simulink model "MiniHR"  (R2023a)
settings: Solver=FixedStepAuto  StartTime=0.0  StopTime=90  RelTol=1e-3
PreLoadFcn:
  | k=0.0001;
InitFcn:
  | k=0.0001;
values from neighbouring files (symbols this model uses):
  X = T(4)    [arm_contr.m]
  Y = T(5)    [arm_contr.m]
  Z = T(6)    [arm_contr.m]
libraries: sm_lib x208, nesl_utility x28, simulink x2
(part 6 of 6)

== system MiniHR/Subsystem/right_foot_y ==
  Visual : sm_lib/Body Elements/File Solid  ExtGeomFileName=小人形关节整合02/meshes/right_foot_y.STL  UnitType=Custom  ExtGeomFileUnits=m  StepReaderType=HEX  ExportConvexHullGeometry=off  InertiaType=Custom  Mass=0.204168570722069  MassUnits=kg  CenterOfMass=[0, 0, 0]  CenterOfMassUnits=m  MomentsOfInertia=[8.623203481057019e-05, 5.19196934874567e-05, 5.75861568294968e-05]  MomentsOfInertiaUnits=kg*m^2  ProductsOfInertia=[-6.07410466001495e-10, -1.79197419171308e-07, -1.07327974268827e-09]  ProductsOfInertiaUnits=kg*m^2  BasedOnType=DensityFromFile  Density=1000  DensityUnits=kg/m^3  DoExposeReferenceFrame=on  SerializedFrames=<Frames/>  GraphicType=FromGeometry  MarkerShape=Sphere  MarkerSize=10  GraphicVisPropType=SimpleVisualProperties  GraphicDiffuseColor=[1.0 0.2 1.0]  GraphicSpecularColor=[0.5 0.5 0.5 1.0]  GraphicAmbientColor=[0.15 0.15 0.15 1.0]  GraphicEmissiveColor=[0.0 0.0 0.0 1.0]  GraphicShininess=75  GraphicOpacity=1
  VisualOriginTransform : sm_lib/Frames and Transforms/Rigid Transform  TranslationMethod=Cartesian  TranslationStandardOffset=0  TranslationStandardOffsetUnits=m  TranslationStandardAxis=+Z  TranslationCartesianOffset=[0, 0, 0]  TranslationCartesianOffsetUnits=m  TranslationROffset=0  TranslationROffsetUnits=m  TranslationZOffset=0  TranslationZOffsetUnits=m  TranslationThetaOffset=0  TranslationThetaOffsetUnits=deg  RotationMethod=RotationSequence  RotationAngleUnits=deg  RotationStandardAxis=+Z  RotationAngle=0.0  RotationArbitraryAxis=[0 0 1]  FollAlignAxisA=+X  BaseAlignAxisA=+Y  FollAlignAxisB=+Y  BaseAlignAxisB=+Z  RotationSequenceAxes=BaseAxes  RotationSequence=XYZ  RotationSequenceAngles=[0, 0, 0]  RotationSequenceAnglesUnits=rad  RotationMatrix=[1 0 0; 0 1 0; 0 0 1]  Quaternion=[1 0 0 0]
  right_foot_x_jo_AxisTransform : sm_lib/Frames and Transforms/Rigid Transform  TranslationMethod=Cartesian  TranslationStandardOffset=0  TranslationStandardOffsetUnits=m  TranslationStandardAxis=+Z  TranslationCartesianOffset=[0, 0, 0]  TranslationCartesianOffsetUnits=m  TranslationROffset=0  TranslationROffsetUnits=m  TranslationZOffset=0  TranslationZOffsetUnits=m  TranslationThetaOffset=0  TranslationThetaOffsetUnits=deg  RotationMethod=ArbitraryAxis  RotationAngleUnits=rad  RotationStandardAxis=+Z  RotationAngle=1.570796326794897  RotationArbitraryAxis=[0, -1, 0]  FollAlignAxisA=+X  BaseAlignAxisA=+Y  FollAlignAxisB=+Y  BaseAlignAxisB=+Z  RotationSequenceAxes=FollowerAxes  RotationSequence=XYX  RotationSequenceAngles=[0 0 0]  RotationSequenceAnglesUnits=deg  RotationMatrix=[1 0 0; 0 1 0; 0 0 1]  Quaternion=[1 0 0 0]
  right_foot_x_jo_OriginTransform : sm_lib/Frames and Transforms/Rigid Transform  TranslationMethod=Cartesian  TranslationStandardOffset=0  TranslationStandardOffsetUnits=m  TranslationStandardAxis=+Z  TranslationCartesianOffset=[0, 0, -0.037]  TranslationCartesianOffsetUnits=m  TranslationROffset=0  TranslationROffsetUnits=m  TranslationZOffset=0  TranslationZOffsetUnits=m  TranslationThetaOffset=0  TranslationThetaOffsetUnits=deg  RotationMethod=RotationSequence  RotationAngleUnits=deg  RotationStandardAxis=+Z  RotationAngle=0.0  RotationArbitraryAxis=[0 0 1]  FollAlignAxisA=+X  BaseAlignAxisA=+Y  FollAlignAxisB=+Y  BaseAlignAxisB=+Z  RotationSequenceAxes=BaseAxes  RotationSequence=XYZ  RotationSequenceAngles=[0, 0, 0]  RotationSequenceAnglesUnits=rad  RotationMatrix=[1 0 0; 0 1 0; 0 0 1]  Quaternion=[1 0 0 0]
  right_foot_y_jo_AxisInvTransform : sm_lib/Frames and Transforms/Rigid Transform  TranslationMethod=Cartesian  TranslationStandardOffset=0  TranslationStandardOffsetUnits=m  TranslationStandardAxis=+Z  TranslationCartesianOffset=[0, 0, 0]  TranslationCartesianOffsetUnits=m  TranslationROffset=0  TranslationROffsetUnits=m  TranslationZOffset=0  TranslationZOffsetUnits=m  TranslationThetaOffset=0  TranslationThetaOffsetUnits=deg  RotationMethod=ArbitraryAxis  RotationAngleUnits=rad  RotationStandardAxis=+Z  RotationAngle=1.570796326794897  RotationArbitraryAxis=[1, 0, 0]  FollAlignAxisA=+X  BaseAlignAxisA=+Y  FollAlignAxisB=+Y  BaseAlignAxisB=+Z  RotationSequenceAxes=FollowerAxes  RotationSequence=XYX  RotationSequenceAngles=[0 0 0]  RotationSequenceAnglesUnits=deg  RotationMatrix=[1 0 0; 0 1 0; 0 0 1]  Quaternion=[1 0 0 0]
  F : PMIOPort  Side=Left
  F1 : PMIOPort  Port=2  Side=Right
  connections:
  VisualOriginTransform/LConn1 -- right_foot_x_jo_OriginTransform/LConn1 -- right_foot_y_jo_AxisInvTransform/LConn1
  Visual/RConn1 -- VisualOriginTransform/RConn1
  right_foot_x_jo_AxisTransform/RConn1 -- F1/RConn1
  right_foot_x_jo_AxisTransform/LConn1 -- right_foot_x_jo_OriginTransform/RConn1
  right_foot_y_jo_AxisInvTransform/RConn1 -- F/RConn1

== system MiniHR/Subsystem/right_hip1 ==
  VisualOriginTransform : sm_lib/Frames and Transforms/Rigid Transform  TranslationMethod=Cartesian  TranslationStandardOffset=0  TranslationStandardOffsetUnits=m  TranslationStandardAxis=+Z  TranslationCartesianOffset=[0, 0, 0]  TranslationCartesianOffsetUnits=m  TranslationROffset=0  TranslationROffsetUnits=m  TranslationZOffset=0  TranslationZOffsetUnits=m  TranslationThetaOffset=0  TranslationThetaOffsetUnits=deg  RotationMethod=RotationSequence  RotationAngleUnits=deg  RotationStandardAxis=+Z  RotationAngle=0.0  RotationArbitraryAxis=[0 0 1]  FollAlignAxisA=+X  BaseAlignAxisA=+Y  FollAlignAxisB=+Y  BaseAlignAxisB=+Z  RotationSequenceAxes=BaseAxes  RotationSequence=XYZ  RotationSequenceAngles=[0, 0, 0]  RotationSequenceAnglesUnits=rad  RotationMatrix=[1 0 0; 0 1 0; 0 0 1]  Quaternion=[1 0 0 0]
  right_hip_pitch : sm_lib/Body Elements/File Solid  ExtGeomFileName=小人形关节整合02/meshes/right_hip1.STL  UnitType=Custom  ExtGeomFileUnits=m  StepReaderType=HEX  ExportConvexHullGeometry=off  InertiaType=Custom  Mass=0.09041873817154029  MassUnits=kg  CenterOfMass=[0, 0, 0]  CenterOfMassUnits=m  MomentsOfInertia=[5.38246679078187e-05, 5.24826042522271e-05, 7.67608010482985e-05]  MomentsOfInertiaUnits=kg*m^2  ProductsOfInertia=[1.82341790079396e-07, -1.67022310989973e-07, -7.72969434280209e-08]  ProductsOfInertiaUnits=kg*m^2  BasedOnType=DensityFromFile  Density=1000  DensityUnits=kg/m^3  DoExposeReferenceFrame=on  SerializedFrames=<Frames/>  GraphicType=FromGeometry  MarkerShape=Sphere  MarkerSize=10  GraphicVisPropType=SimpleVisualProperties  GraphicDiffuseColor=[0.898039215686275, 0.917647058823529, 0.929411764705882]  GraphicSpecularColor=[0.5 0.5 0.5 1.0]  GraphicAmbientColor=[0.15 0.15 0.15 1.0]  GraphicEmissiveColor=[0.0 0.0 0.0 1.0]  GraphicShininess=75  GraphicOpacity=1
  right_hip_pitch_AxisInvTransform : sm_lib/Frames and Transforms/Rigid Transform  TranslationMethod=Cartesian  TranslationStandardOffset=0  TranslationStandardOffsetUnits=m  TranslationStandardAxis=+Z  TranslationCartesianOffset=[0, 0, 0]  TranslationCartesianOffsetUnits=m  TranslationROffset=0  TranslationROffsetUnits=m  TranslationZOffset=0  TranslationZOffsetUnits=m  TranslationThetaOffset=0  TranslationThetaOffsetUnits=deg  RotationMethod=ArbitraryAxis  RotationAngleUnits=rad  RotationStandardAxis=+Z  RotationAngle=1.570796326794897  RotationArbitraryAxis=[-1, 0, 0]  FollAlignAxisA=+X  BaseAlignAxisA=+Y  FollAlignAxisB=+Y  BaseAlignAxisB=+Z  RotationSequenceAxes=FollowerAxes  RotationSequence=XYX  RotationSequenceAngles=[0 0 0]  RotationSequenceAnglesUnits=deg  RotationMatrix=[1 0 0; 0 1 0; 0 0 1]  Quaternion=[1 0 0 0]
  right_hip_roll_AxisTransform : sm_lib/Frames and Transforms/Rigid Transform  TranslationMethod=Cartesian  TranslationStandardOffset=0  TranslationStandardOffsetUnits=m  TranslationStandardAxis=+Z  TranslationCartesianOffset=[0, 0, 0]  TranslationCartesianOffsetUnits=m  TranslationROffset=0  TranslationROffsetUnits=m  TranslationZOffset=0  TranslationZOffsetUnits=m  TranslationThetaOffset=0  TranslationThetaOffsetUnits=deg  RotationMethod=ArbitraryAxis  RotationAngleUnits=rad  RotationStandardAxis=+Z  RotationAngle=1.570796326794897  RotationArbitraryAxis=[-0, 1, 0]  FollAlignAxisA=+X  BaseAlignAxisA=+Y  FollAlignAxisB=+Y  BaseAlignAxisB=+Z  RotationSequenceAxes=FollowerAxes  RotationSequence=XYX  RotationSequenceAngles=[0 0 0]  RotationSequenceAnglesUnits=deg  RotationMatrix=[1 0 0; 0 1 0; 0 0 1]  Quaternion=[1 0 0 0]
  right_hip_roll_OriginTransform : sm_lib/Frames and Transforms/Rigid Transform  TranslationMethod=Cartesian  TranslationStandardOffset=0  TranslationStandardOffsetUnits=m  TranslationStandardAxis=+Z  TranslationCartesianOffset="[ -0.00185,  -0.0055,   -0.024]"  TranslationCartesianOffsetUnits=m  TranslationROffset=0  TranslationROffsetUnits=m  TranslationZOffset=0  TranslationZOffsetUnits=m  TranslationThetaOffset=0  TranslationThetaOffsetUnits=deg  RotationMethod=RotationSequence  RotationAngleUnits=deg  RotationStandardAxis=+Z  RotationAngle=0.0  RotationArbitraryAxis=[0 0 1]  FollAlignAxisA=+X  BaseAlignAxisA=+Y  FollAlignAxisB=+Y  BaseAlignAxisB=+Z  RotationSequenceAxes=BaseAxes  RotationSequence=XYZ  RotationSequenceAngles=[0, 0, 0]  RotationSequenceAnglesUnits=rad  RotationMatrix=[1 0 0; 0 1 0; 0 0 1]  Quaternion=[1 0 0 0]
  F : PMIOPort  Side=Left
  F1 : PMIOPort  Port=2  Side=Right
  connections:
  VisualOriginTransform/LConn1 -- right_hip_pitch_AxisInvTransform/LConn1 -- right_hip_roll_OriginTransform/LConn1
  right_hip_pitch/RConn1 -- VisualOriginTransform/RConn1
  right_hip_pitch_AxisInvTransform/RConn1 -- F/RConn1
  right_hip_roll_AxisTransform/RConn1 -- F1/RConn1
  right_hip_roll_AxisTransform/LConn1 -- right_hip_roll_OriginTransform/RConn1

== system MiniHR/Subsystem/right_hip2 ==
  VisualOriginTransform : sm_lib/Frames and Transforms/Rigid Transform  TranslationMethod=Cartesian  TranslationStandardOffset=0  TranslationStandardOffsetUnits=m  TranslationStandardAxis=+Z  TranslationCartesianOffset=[0, 0, 0]  TranslationCartesianOffsetUnits=m  TranslationROffset=0  TranslationROffsetUnits=m  TranslationZOffset=0  TranslationZOffsetUnits=m  TranslationThetaOffset=0  TranslationThetaOffsetUnits=deg  RotationMethod=RotationSequence  RotationAngleUnits=deg  RotationStandardAxis=+Z  RotationAngle=0.0  RotationArbitraryAxis=[0 0 1]  FollAlignAxisA=+X  BaseAlignAxisA=+Y  FollAlignAxisB=+Y  BaseAlignAxisB=+Z  RotationSequenceAxes=BaseAxes  RotationSequence=XYZ  RotationSequenceAngles=[0, 0, 0]  RotationSequenceAnglesUnits=rad  RotationMatrix=[1 0 0; 0 1 0; 0 0 1]  Quaternion=[1 0 0 0]
  right_hip_roll : sm_lib/Body Elements/File Solid  ExtGeomFileName=小人形关节整合02/meshes/right_hip2.STL  UnitType=Custom  ExtGeomFileUnits=m  StepReaderType=HEX  ExportConvexHullGeometry=off  InertiaType=Custom  Mass=0.164190861193546  MassUnits=kg  CenterOfMass=[0, 0, 0]  CenterOfMassUnits=m  MomentsOfInertia=[5.215641323237e-05, 2.61205317951127e-05, 5.86715753089718e-05]  MomentsOfInertiaUnits=kg*m^2  ProductsOfInertia=[-2.208848562922e-08, 1.31358874032874e-07, -1.19039463273149e-08]  ProductsOfInertiaUnits=kg*m^2  BasedOnType=DensityFromFile  Density=1000  DensityUnits=kg/m^3  DoExposeReferenceFrame=on  SerializedFrames=<Frames/>  GraphicType=FromGeometry  MarkerShape=Sphere  MarkerSize=10  GraphicVisPropType=SimpleVisualProperties  GraphicDiffuseColor=[1.0 0.2 1.0]  GraphicSpecularColor=[0.5 0.5 0.5 1.0]  GraphicAmbientColor=[0.15 0.15 0.15 1.0]  GraphicEmissiveColor=[0.0 0.0 0.0 1.0]  GraphicShininess=75  GraphicOpacity=1
  right_hip_roll_AxisInvTransform : sm_lib/Frames and Transforms/Rigid Transform  TranslationMethod=Cartesian  TranslationStandardOffset=0  TranslationStandardOffsetUnits=m  TranslationStandardAxis=+Z  TranslationCartesianOffset=[0, 0, 0]  TranslationCartesianOffsetUnits=m  TranslationROffset=0  TranslationROffsetUnits=m  TranslationZOffset=0  TranslationZOffsetUnits=m  TranslationThetaOffset=0  TranslationThetaOffsetUnits=deg  RotationMethod=ArbitraryAxis  RotationAngleUnits=rad  RotationStandardAxis=+Z  RotationAngle=1.570796326794897  RotationArbitraryAxis=[-0, 1, 0]  FollAlignAxisA=+X  BaseAlignAxisA=+Y  FollAlignAxisB=+Y  BaseAlignAxisB=+Z  RotationSequenceAxes=FollowerAxes  RotationSequence=XYX  RotationSequenceAngles=[0 0 0]  RotationSequenceAnglesUnits=deg  RotationMatrix=[1 0 0; 0 1 0; 0 0 1]  Quaternion=[1 0 0 0]
  right_hip_yaw_AxisTransform : sm_lib/Frames and Transforms/Rigid Transform  TranslationMethod=Cartesian  TranslationStandardOffset=0  TranslationStandardOffsetUnits=m  TranslationStandardAxis=+Z  TranslationCartesianOffset=[0, 0, 0]  TranslationCartesianOffsetUnits=m  TranslationROffset=0  TranslationROffsetUnits=m  TranslationZOffset=0  TranslationZOffsetUnits=m  TranslationThetaOffset=0  TranslationThetaOffsetUnits=deg  RotationMethod=ArbitraryAxis  RotationAngleUnits=rad  RotationStandardAxis=+Z  RotationAngle=3.141592653589793  RotationArbitraryAxis=[1, 0, 0]  FollAlignAxisA=+X  BaseAlignAxisA=+Y  FollAlignAxisB=+Y  BaseAlignAxisB=+Z  RotationSequenceAxes=FollowerAxes  RotationSequence=XYX  RotationSequenceAngles=[0 0 0]  RotationSequenceAnglesUnits=deg  RotationMatrix=[1 0 0; 0 1 0; 0 0 1]  Quaternion=[1 0 0 0]
  right_hip_yaw_OriginTransform : sm_lib/Frames and Transforms/Rigid Transform  TranslationMethod=Cartesian  TranslationStandardOffset=0  TranslationStandardOffsetUnits=m  TranslationStandardAxis=+Z  TranslationCartesianOffset="[0         ,0.0055,  -0.02315]"  TranslationCartesianOffsetUnits=m  TranslationROffset=0  TranslationROffsetUnits=m  TranslationZOffset=0  TranslationZOffsetUnits=m  TranslationThetaOffset=0  TranslationThetaOffsetUnits=deg  RotationMethod=RotationSequence  RotationAngleUnits=deg  RotationStandardAxis=+Z  RotationAngle=0.0  RotationArbitraryAxis=[0 0 1]  FollAlignAxisA=+X  BaseAlignAxisA=+Y  FollAlignAxisB=+Y  BaseAlignAxisB=+Z  RotationSequenceAxes=BaseAxes  RotationSequence=XYZ  RotationSequenceAngles=[0, 0, 0]  RotationSequenceAnglesUnits=rad  RotationMatrix=[1 0 0; 0 1 0; 0 0 1]  Quaternion=[1 0 0 0]
  F : PMIOPort  Side=Left
  F1 : PMIOPort  Port=2  Side=Right
  connections:
  right_hip_roll_AxisInvTransform/LConn1 -- VisualOriginTransform/LConn1 -- right_hip_yaw_OriginTransform/LConn1
  right_hip_roll/RConn1 -- VisualOriginTransform/RConn1
  right_hip_roll_AxisInvTransform/RConn1 -- F/RConn1
  right_hip_yaw_AxisTransform/RConn1 -- F1/RConn1
  right_hip_yaw_AxisTransform/LConn1 -- right_hip_yaw_OriginTransform/RConn1

== system MiniHR/Subsystem/right_hip3 ==
  VisualOriginTransform : sm_lib/Frames and Transforms/Rigid Transform  TranslationMethod=Cartesian  TranslationStandardOffset=0  TranslationStandardOffsetUnits=m  TranslationStandardAxis=+Z  TranslationCartesianOffset=[0, 0, 0]  TranslationCartesianOffsetUnits=m  TranslationROffset=0  TranslationROffsetUnits=m  TranslationZOffset=0  TranslationZOffsetUnits=m  TranslationThetaOffset=0  TranslationThetaOffsetUnits=deg  RotationMethod=RotationSequence  RotationAngleUnits=deg  RotationStandardAxis=+Z  RotationAngle=0.0  RotationArbitraryAxis=[0 0 1]  FollAlignAxisA=+X  BaseAlignAxisA=+Y  FollAlignAxisB=+Y  BaseAlignAxisB=+Z  RotationSequenceAxes=BaseAxes  RotationSequence=XYZ  RotationSequenceAngles=[0, 0, 0]  RotationSequenceAnglesUnits=rad  RotationMatrix=[1 0 0; 0 1 0; 0 0 1]  Quaternion=[1 0 0 0]
  right_hip_yaw : sm_lib/Body Elements/File Solid  ExtGeomFileName=小人形关节整合02/meshes/right_hip3.STL  UnitType=Custom  ExtGeomFileUnits=m  StepReaderType=HEX  ExportConvexHullGeometry=off  InertiaType=Custom  Mass=0.47372999581153  MassUnits=kg  CenterOfMass=[0, 0, 0]  CenterOfMassUnits=m  MomentsOfInertia=[0.000481949796096193, 0.000388294415269902, 0.000181274621011488]  MomentsOfInertiaUnits=kg*m^2  ProductsOfInertia=[-1.42075949096599e-05, 1.278669641739e-05, -3.81271886359838e-06]  ProductsOfInertiaUnits=kg*m^2  BasedOnType=DensityFromFile  Density=1000  DensityUnits=kg/m^3  DoExposeReferenceFrame=on  SerializedFrames=<Frames/>  GraphicType=FromGeometry  MarkerShape=Sphere  MarkerSize=10  GraphicVisPropType=SimpleVisualProperties  GraphicDiffuseColor=[0.898039215686275, 0.917647058823529, 0.929411764705882]  GraphicSpecularColor=[0.5 0.5 0.5 1.0]  GraphicAmbientColor=[0.15 0.15 0.15 1.0]  GraphicEmissiveColor=[0.0 0.0 0.0 1.0]  GraphicShininess=75  GraphicOpacity=1
  right_hip_yaw_AxisInvTransform : sm_lib/Frames and Transforms/Rigid Transform  TranslationMethod=Cartesian  TranslationStandardOffset=0  TranslationStandardOffsetUnits=m  TranslationStandardAxis=+Z  TranslationCartesianOffset=[0, 0, 0]  TranslationCartesianOffsetUnits=m  TranslationROffset=0  TranslationROffsetUnits=m  TranslationZOffset=0  TranslationZOffsetUnits=m  TranslationThetaOffset=0  TranslationThetaOffsetUnits=deg  RotationMethod=ArbitraryAxis  RotationAngleUnits=rad  RotationStandardAxis=+Z  RotationAngle=3.141592653589793  RotationArbitraryAxis=[1, 0, 0]  FollAlignAxisA=+X  BaseAlignAxisA=+Y  FollAlignAxisB=+Y  BaseAlignAxisB=+Z  RotationSequenceAxes=FollowerAxes  RotationSequence=XYX  RotationSequenceAngles=[0 0 0]  RotationSequenceAnglesUnits=deg  RotationMatrix=[1 0 0; 0 1 0; 0 0 1]  Quaternion=[1 0 0 0]
  right_knee_jo_AxisTransform : sm_lib/Frames and Transforms/Rigid Transform  TranslationMethod=Cartesian  TranslationStandardOffset=0  TranslationStandardOffsetUnits=m  TranslationStandardAxis=+Z  TranslationCartesianOffset=[0, 0, 0]  TranslationCartesianOffsetUnits=m  TranslationROffset=0  TranslationROffsetUnits=m  TranslationZOffset=0  TranslationZOffsetUnits=m  TranslationThetaOffset=0  TranslationThetaOffsetUnits=deg  RotationMethod=ArbitraryAxis  RotationAngleUnits=rad  RotationStandardAxis=+Z  RotationAngle=1.570796326794897  RotationArbitraryAxis=[1, 0, 0]  FollAlignAxisA=+X  BaseAlignAxisA=+Y  FollAlignAxisB=+Y  BaseAlignAxisB=+Z  RotationSequenceAxes=FollowerAxes  RotationSequence=XYX  RotationSequenceAngles=[0 0 0]  RotationSequenceAnglesUnits=deg  RotationMatrix=[1 0 0; 0 1 0; 0 0 1]  Quaternion=[1 0 0 0]
  right_knee_jo_OriginTransform : sm_lib/Frames and Transforms/Rigid Transform  TranslationMethod=Cartesian  TranslationStandardOffset=0  TranslationStandardOffsetUnits=m  TranslationStandardAxis=+Z  TranslationCartesianOffset=[-0.0045,0, -0.128]  TranslationCartesianOffsetUnits=m  TranslationROffset=0  TranslationROffsetUnits=m  TranslationZOffset=0  TranslationZOffsetUnits=m  TranslationThetaOffset=0  TranslationThetaOffsetUnits=deg  RotationMethod=RotationSequence  RotationAngleUnits=deg  RotationStandardAxis=+Z  RotationAngle=0.0  RotationArbitraryAxis=[0 0 1]  FollAlignAxisA=+X  BaseAlignAxisA=+Y  FollAlignAxisB=+Y  BaseAlignAxisB=+Z  RotationSequenceAxes=BaseAxes  RotationSequence=XYZ  RotationSequenceAngles=[0, 0, 0]  RotationSequenceAnglesUnits=rad  RotationMatrix=[1 0 0; 0 1 0; 0 0 1]  Quaternion=[1 0 0 0]
  F : PMIOPort  Side=Left
  F1 : PMIOPort  Port=2  Side=Right
  connections:
  VisualOriginTransform/LConn1 -- right_hip_yaw_AxisInvTransform/LConn1 -- right_knee_jo_OriginTransform/LConn1
  right_hip_yaw/RConn1 -- VisualOriginTransform/RConn1
  right_hip_yaw_AxisInvTransform/RConn1 -- F/RConn1
  right_knee_jo_AxisTransform/RConn1 -- F1/RConn1
  right_knee_jo_AxisTransform/LConn1 -- right_knee_jo_OriginTransform/RConn1

== system MiniHR/Subsystem/right_knee ==
  Visual : sm_lib/Body Elements/File Solid  ExtGeomFileName=小人形关节整合02/meshes/right_knee.STL  UnitType=Custom  ExtGeomFileUnits=m  StepReaderType=HEX  ExportConvexHullGeometry=off  InertiaType=Custom  Mass=0.373447646908613  MassUnits=kg  CenterOfMass=[0, 0, 0]  CenterOfMassUnits=m  MomentsOfInertia=[0.000429162766551639, 0.000322151019554768, 0.000158922625277449]  MomentsOfInertiaUnits=kg*m^2  ProductsOfInertia=[-4.58205901445265e-06, 1.62879548340809e-05, 1.60301527579783e-06]  ProductsOfInertiaUnits=kg*m^2  BasedOnType=DensityFromFile  Density=1000  DensityUnits=kg/m^3  DoExposeReferenceFrame=on  SerializedFrames=<Frames/>  GraphicType=FromGeometry  MarkerShape=Sphere  MarkerSize=10  GraphicVisPropType=SimpleVisualProperties  GraphicDiffuseColor=[0.898039215686275, 0.917647058823529, 0.929411764705882]  GraphicSpecularColor=[0.5 0.5 0.5 1.0]  GraphicAmbientColor=[0.15 0.15 0.15 1.0]  GraphicEmissiveColor=[0.0 0.0 0.0 1.0]  GraphicShininess=75  GraphicOpacity=1
  VisualOriginTransform : sm_lib/Frames and Transforms/Rigid Transform  TranslationMethod=Cartesian  TranslationStandardOffset=0  TranslationStandardOffsetUnits=m  TranslationStandardAxis=+Z  TranslationCartesianOffset=[0, 0, 0]  TranslationCartesianOffsetUnits=m  TranslationROffset=0  TranslationROffsetUnits=m  TranslationZOffset=0  TranslationZOffsetUnits=m  TranslationThetaOffset=0  TranslationThetaOffsetUnits=deg  RotationMethod=RotationSequence  RotationAngleUnits=deg  RotationStandardAxis=+Z  RotationAngle=0.0  RotationArbitraryAxis=[0 0 1]  FollAlignAxisA=+X  BaseAlignAxisA=+Y  FollAlignAxisB=+Y  BaseAlignAxisB=+Z  RotationSequenceAxes=BaseAxes  RotationSequence=XYZ  RotationSequenceAngles=[0, 0, 0]  RotationSequenceAnglesUnits=rad  RotationMatrix=[1 0 0; 0 1 0; 0 0 1]  Quaternion=[1 0 0 0]
  right_foot_y_jo_AxisTransform : sm_lib/Frames and Transforms/Rigid Transform  TranslationMethod=Cartesian  TranslationStandardOffset=0  TranslationStandardOffsetUnits=m  TranslationStandardAxis=+Z  TranslationCartesianOffset=[0, 0, 0]  TranslationCartesianOffsetUnits=m  TranslationROffset=0  TranslationROffsetUnits=m  TranslationZOffset=0  TranslationZOffsetUnits=m  TranslationThetaOffset=0  TranslationThetaOffsetUnits=deg  RotationMethod=ArbitraryAxis  RotationAngleUnits=rad  RotationStandardAxis=+Z  RotationAngle=1.570796326794897  RotationArbitraryAxis=[1, 0, 0]  FollAlignAxisA=+X  BaseAlignAxisA=+Y  FollAlignAxisB=+Y  BaseAlignAxisB=+Z  RotationSequenceAxes=FollowerAxes  RotationSequence=XYX  RotationSequenceAngles=[0 0 0]  RotationSequenceAnglesUnits=deg  RotationMatrix=[1 0 0; 0 1 0; 0 0 1]  Quaternion=[1 0 0 0]
  right_foot_y_jo_OriginTransform : sm_lib/Frames and Transforms/Rigid Transform  TranslationMethod=Cartesian  TranslationStandardOffset=0  TranslationStandardOffsetUnits=m  TranslationStandardAxis=+Z  TranslationCartesianOffset=[0.008, 0, -0.118]  TranslationCartesianOffsetUnits=m  TranslationROffset=0  TranslationROffsetUnits=m  TranslationZOffset=0  TranslationZOffsetUnits=m  TranslationThetaOffset=0  TranslationThetaOffsetUnits=deg  RotationMethod=RotationSequence  RotationAngleUnits=deg  RotationStandardAxis=+Z  RotationAngle=0.0  RotationArbitraryAxis=[0 0 1]  FollAlignAxisA=+X  BaseAlignAxisA=+Y  FollAlignAxisB=+Y  BaseAlignAxisB=+Z  RotationSequenceAxes=BaseAxes  RotationSequence=XYZ  RotationSequenceAngles=[0, 0, 0]  RotationSequenceAnglesUnits=rad  RotationMatrix=[1 0 0; 0 1 0; 0 0 1]  Quaternion=[1 0 0 0]
  right_knee_jo_AxisInvTransform : sm_lib/Frames and Transforms/Rigid Transform  TranslationMethod=Cartesian  TranslationStandardOffset=0  TranslationStandardOffsetUnits=m  TranslationStandardAxis=+Z  TranslationCartesianOffset=[0, 0, 0]  TranslationCartesianOffsetUnits=m  TranslationROffset=0  TranslationROffsetUnits=m  TranslationZOffset=0  TranslationZOffsetUnits=m  TranslationThetaOffset=0  TranslationThetaOffsetUnits=deg  RotationMethod=ArbitraryAxis  RotationAngleUnits=rad  RotationStandardAxis=+Z  RotationAngle=1.570796326794897  RotationArbitraryAxis=[1, 0, 0]  FollAlignAxisA=+X  BaseAlignAxisA=+Y  FollAlignAxisB=+Y  BaseAlignAxisB=+Z  RotationSequenceAxes=FollowerAxes  RotationSequence=XYX  RotationSequenceAngles=[0 0 0]  RotationSequenceAnglesUnits=deg  RotationMatrix=[1 0 0; 0 1 0; 0 0 1]  Quaternion=[1 0 0 0]
  F : PMIOPort  Side=Left
  F1 : PMIOPort  Port=2  Side=Right
  connections:
  VisualOriginTransform/LConn1 -- right_foot_y_jo_OriginTransform/LConn1 -- right_knee_jo_AxisInvTransform/LConn1
  Visual/RConn1 -- VisualOriginTransform/RConn1
  right_foot_y_jo_AxisTransform/RConn1 -- F1/RConn1
  right_foot_y_jo_AxisTransform/LConn1 -- right_foot_y_jo_OriginTransform/RConn1
  right_knee_jo_AxisInvTransform/RConn1 -- F/RConn1

== matlab function MiniHR/Subsystem/If Action Subsystem/MATLAB Function ==
  data: q0 input; q output; q1 input; qd0 input; qd1 input; T input; t input
function q  = Cubic_polynomial_interpolation(q0, q1, qd0, qd1, T, t)
    % 给定初末位置、速度、总时间，返回三次插值后，在时间t（0<t<T）的位置、速度、加速度，t也可以是时间序列
    A = [  0  ,  0 , 0, 1;
         T^3  , T^2, T, 1;
         0    ,  0 , 1, 0;
         3*T^2, 2*T, 1, 0];
    
    B = [q0; q1; qd0; qd1];
    
    % 求解系数矩阵
    p = A \ B;

    % 计算位置、速度、加速度
    q = p(1, :)' * t.^3 + p(2, :)' * t.^2 + p(3, :)' * t + p(4, :)';
    qd = 3 * p(1, :)' * t.^2 + 2 * p(2, :)' * t + p(3, :)';
    qdd = 6 * p(1, :)' * t + 2 * p(2, :)';

end

== matlab function MiniHR/Subsystem/If Action Subsystem/MATLAB Function1 ==
  data: z input; L_Hip_Yaw output; lr input; L_Hip_Roll output; L_Hip_Pitch output; L_knee output; L_Ankle_Pitch output; L_Ankle_Roll output
function [L_Hip_Yaw,L_Hip_Roll,L_Hip_Pitch,L_knee,L_Ankle_Pitch,L_Ankle_Roll]=ik(z,lr)
%腿部逆运动学
%已知质心位置pc，脚底中心位置pf，计算左腿关节角度
%输出结果为从上到下依次关节角度，默认膝关节前弯


pc=[0,0,z];
pf=[0.00055,0.095,0];
if lr==1 %左腿
    phip=pc+[-0.0011  0.095  -0.013327] ;%髋关节位置  [-0.0011  0.095  -0.013327]

    phip2_roll=phip+[-0.00185, 0,   -0.024];
    knee=phip2_roll+[ 0,        -0.00525,  -0.02315]+[ -0.0045,   0.0000,  -0.128];
     pankle=pf-[ 0, 0, -0.037];

else %右腿
    phip=pc+[-0.0011 -0.095 -0.013327]; %髋关节位置 [-0.0011 -0.095 -0.013327 ]
    phip2_roll=phip+[ -0.00185,  0,   -0.024];

    knee=phip2_roll+[ 0         ,0.00525,  -0.02315]+[  -0.0045,   0.0000,  -0.128];
    pankle=pf-[ 0, 0, -0.037];
end

%% 三杆长度计算
 l2 =0.1183;
 l1=norm(phip-knee);

 %踝关节位置   
Lleg = norm(pankle-phip)+3.813e-04; %腿长  
Rleg=norm([phip2_roll(2),phip2_roll(3)]-[pf(2),pf(3)]);

%膝关节角度
  % L_knee1=pi-2*asin(Lleg);  % Π -2

%% 三角形几何解
% L_knee=(-acos((l1^2+l2^2-Lleg^2)/(2*l1*l2))+pi);
% L_Ankle_Pitch=-asin((l1*sin(pi-L_knee)/Lleg));

L_knee = (-acos(max(-1, min(1, (l1^2 + l2^2 - Lleg^2) / (2 * l1 * l2)))) + pi);
% L_Ankle_Pitch =asin((knee(1)-pankle(1)+0.008)/l2)+0.5*L_knee;
 % L_Ankle_Pitch=-asin(max(-1,min(1,(pankle(1)-phip(1)/Lleg ))));+asin((abs(pankle(1)-phip(1)-0.00165)/Lleg));asin(abs(knee(1)-pankle(1))/l2);
% L_Hip_Pitch=L_knee-abs(asin(max(-1, min(1, (l1 * sin(pi - L_knee) / Lleg)))))+asin(abs(pankle(1)-phip(1)-0.00165)/Lleg);
L_Hip_Pitch=acos(max(-1, min(1, (l1^2 + Lleg^2 - l2^2) / (2 * l1 * Lleg))))+atan((pankle(1)-phip(1)-0.00055)/(-pankle(3)+phip(3)));
L_Ankle_Pitch =L_knee-L_Hip_Pitch;

%% 侧摆
% L_Hip_Roll=-asin((abs(pf(2)-phip2_roll(2))-0.0055)/norm(phip2_roll(2:3)-pf(2:3)));
L_Hip_Roll=asin((phip2_roll(2)-pf(2))/Rleg);
L_Ankle_Roll=-L_Hip_Roll;
L_Hip_Yaw=0;

end

== matlab function MiniHR/Subsystem/If Action Subsystem/MATLAB Function2 ==
  data: z input; L_Hip_Yaw output; lr input; L_Hip_Roll output; L_Hip_Pitch output; L_knee output; L_Ankle_Pitch output; L_Ankle_Roll output
function [L_Hip_Yaw,L_Hip_Roll,L_Hip_Pitch,L_knee,L_Ankle_Pitch,L_Ankle_Roll]=ik(z,lr)
%腿部逆运动学
%已知质心位置pc，脚底中心位置pf，计算左腿关节角度
%输出结果为从上到下依次关节角度，默认膝关节前弯


pc=[0,0,z];
pf=[0.00055,-0.095,0];
if lr==1 %左腿
    phip=pc+[-0.0011  0.095  -0.013327] ;%髋关节位置  [-0.0011  0.095  -0.013327]

    phip2_roll=phip+[-0.00185, 0,   -0.024];
    knee=phip2_roll+[ 0,        -0.00525,  -0.02315]+[ -0.0045,   0.0000,  -0.128];
     pankle=pf-[ 0, 0, -0.037];

else %右腿
    phip=pc+[-0.0011 -0.095 -0.013327]; %髋关节位置 [-0.0011 -0.095 -0.013327 ]
    phip2_roll=phip+[ -0.00185,  0,   -0.024];

    knee=phip2_roll+[ 0         ,0.00525,  -0.02315]+[  -0.0045,   0.0000,  -0.128];
    pankle=pf-[ 0, 0, -0.037];
end

%% 三杆长度计算
 l2 =0.1183;
 l1=norm(phip-knee);

 %踝关节位置   
Lleg = norm(pankle-phip)+3.813e-04; %腿长  
Rleg=norm([phip2_roll(2),phip2_roll(3)]-[pf(2),pf(3)]);

%膝关节角度
  % L_knee1=pi-2*asin(Lleg);  % Π -2

%% 三角形几何解
% L_knee=(-acos((l1^2+l2^2-Lleg^2)/(2*l1*l2))+pi);
% L_Ankle_Pitch=-asin((l1*sin(pi-L_knee)/Lleg));

L_knee = (-acos(max(-1, min(1, (l1^2 + l2^2 - Lleg^2) / (2 * l1 * l2)))) + pi);
% L_Ankle_Pitch =asin((knee(1)-pankle(1)+0.008)/l2)+0.5*L_knee;
 % L_Ankle_Pitch=-asin(max(-1,min(1,(pankle(1)-phip(1)/Lleg ))));+asin((abs(pankle(1)-phip(1)-0.00165)/Lleg));asin(abs(knee(1)-pankle(1))/l2);
% L_Hip_Pitch=L_knee-abs(asin(max(-1, min(1, (l1 * sin(pi - L_knee) / Lleg)))))+asin(abs(pankle(1)-phip(1)-0.00165)/Lleg);
L_Hip_Pitch=acos(max(-1, min(1, (l1^2 + Lleg^2 - l2^2) / (2 * l1 * Lleg))))+atan((pankle(1)-phip(1)-0.00055)/(-pankle(3)+phip(3)));
L_Ankle_Pitch =L_knee-L_Hip_Pitch;

%% 侧摆
% L_Hip_Roll=-asin((abs(pf(2)-phip2_roll(2))-0.0055)/norm(phip2_roll(2:3)-pf(2:3)));
L_Hip_Roll=asin((phip2_roll(2)-pf(2))/Rleg);
L_Ankle_Roll=-L_Hip_Roll;
L_Hip_Yaw=0;

end
